simulink model "Switch_Block_2"  (R2021a)
settings: Solver=VariableStepAuto  StartTime=0.0  StopTime=10.0  RelTol=1e-3
settings Model: Creator=lenovo  LastModifiedBy=lenovo

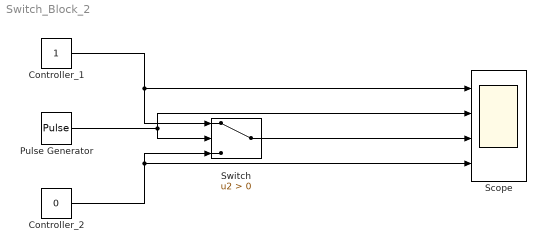
== system Switch_Block_2 ==
  Controller_1 : Constant
  Controller_2 : Constant  Value=0
  Pulse Generator : DiscretePulseGenerator  PulseType=Time based  Period=1  PulseWidth=25
  Scope : Scope  NumInputPorts=4
  Switch : Switch  Criteria=u2 > Threshold
  wires:
  Controller_1/1 -> Switch/1, Scope/1
  Controller_2/1 -> Scope/4, Switch/3
  Pulse Generator/1 -> Switch/2, Scope/2
  Switch/1 -> Scope/3
